simulink model "p2_d_sim"  (R2019a)
settings: Solver=VariableStepAuto  StartTime=0.0  StopTime=200  RelTol=1e-3
values from neighbouring files (symbols this model uses):
  a_phi1 = 2.87    [p2_d.m]    (also in p2_e.m)
  a_phi2 = -0.65    [p2_d.m]    (also in p2_e.m)
  k_dphi = k_d_phi    [p2_d.m]    (also in p2_e.m)
  k_g = g/V_g    (= 0.0608896551724)    [p2_d.m]    (also in p2_e.m)
  k_iphi = k_i_phi    (= -0.6)    [p2_d.m]    (also in p2_e.m)
  k_ix = k_i_chi    [p2_d.m]    (also in p2_e.m)
  k_pphi = k_p_phi    [p2_d.m]    (also in p2_e.m)
  k_px = k_p_chi    [p2_d.m]    (also in p2_e.m)
undefined symbols (not defined in the file or in its folder): sigbuilder_block
libraries: simulink_extras x2
settings Model: Creator=lenovo  LastModifiedBy=zhy

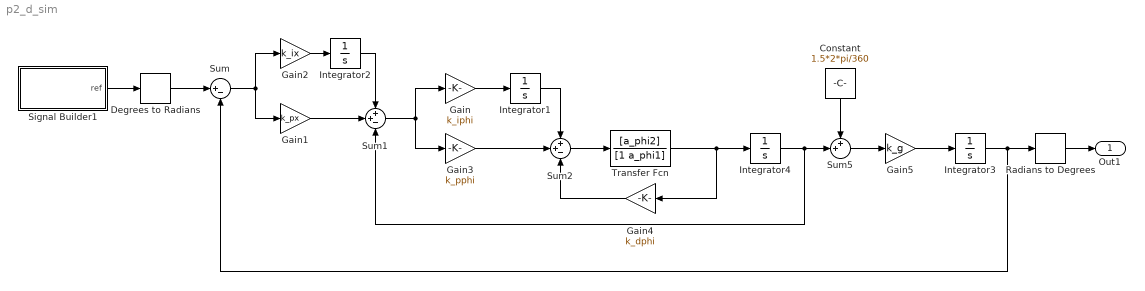
== system p2_d_sim ==
  Constant : Constant  Value=1.5*2*pi/360
  Degrees to Radians : simulink_extras/Transformations/Degrees to Radians
  Gain : Gain  Gain=k_iphi
  Gain1 : Gain  Gain=k_px
  Gain2 : Gain  Gain=k_ix
  Gain3 : Gain  Gain=k_pphi
  Gain4 : Gain  Gain=k_dphi
  Gain5 : Gain  Gain=k_g
  Integrator{1..4} (4 alike) : Integrator
  Radians to Degrees : simulink_extras/Transformations/Radians to Degrees
  Signal Builder1 : Subsystem  Tag=STV Subsys  LoadFcn=sigbuilder_block('load');  StartFcn=sigbuilder_block('start');  StopFcn=sigbuilder_block('stop');  ClipboardFcn=sigbuilder_block('clipboard');  mask(Sigbuilder block){tuvar=[0:10]}
      mask help: Simulink:masks:SigbuilderBlock_MD
      mask init:
      | if ~strcmp(get_param(bdroot(gcbh),'SimulationStatus'),'stopped') tuvar = sigbuilder_block('maskInit'); end
      settings: CopyFcn=sigbuilder_block('copy');  DeleteFcn=sigbuilder_block('delete');  ModelCloseFcn=sigbuilder_block('modelClose');  PreSaveFcn=sigbuilder_block('preSave');  PauseFcn=sigbuilder_block('pause');  ContinueFcn=sigbuilder_block('continue');  NameChangeFcn=sigbuilder_block('namechange');  OpenFcn=sigbuilder_block('open',[411 163.2 550.8 400.2 ]);  CloseFcn=sigbuilder_block('close');
      mask Display: plot(0, 0, 100, 100,[2, 2, 32, 32, 2], [68, 8, 8, 68, 68],[32, 2], [38, 38], [32, 19, 2],[53, 60, 44], [32, 17, 17, 2],[16, 16, 31, 31]);txt = getActiveGroup(gcbh);text(2, 100, txt,'verticalAlignment', 'top');
  Sum : Sum  Inputs=|+-
  Sum1 : Sum  Inputs=++-
  Sum2 : Sum  Inputs=++-
  Sum5 : Sum  Inputs=++|
  Transfer Fcn : TransferFcn  Numerator=[a_phi2]  Denominator=[1 a_phi1]
  Out1 : Outport
  wires:
  Sum/1 -> Gain1/1, Gain2/1
  Sum1/1 -> Gain3/1, Gain/1
  Sum5/1 -> Gain5/1
  Degrees to Radians/1 -> Sum/1
  Gain2/1 -> Integrator2/1
  Integrator2/1 -> Sum1/1
  Gain1/1 -> Sum1/2
  Gain/1 -> Integrator1/1
  Gain3/1 -> Sum2/2
  Transfer Fcn/1 -> Gain4/1, Integrator4/1
  Integrator4/1 -> Sum5/2, Sum1/3
  Constant/1 -> Sum5/1
  Integrator3/1 -> Radians to Degrees/1, Sum/2
  Gain5/1 -> Integrator3/1
  Signal Builder1/1(ref) -> Degrees to Radians/1
  Sum2/1 -> Transfer Fcn/1
  Gain4/1 -> Sum2/3
  Integrator1/1 -> Sum2/1
  Radians to Degrees/1 -> Out1/1

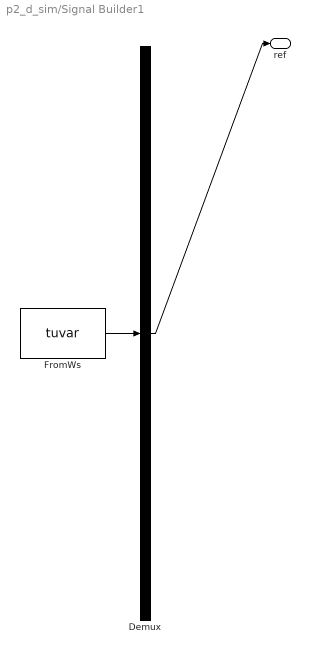
== system p2_d_sim/Signal Builder1 ==
  Demux : Demux  Tag=STV Demux  Outputs=1
  FromWs : FromWorkspace  Tag=STV FromWs  VariableName=tuvar  SampleTime=0
      SigBuilderData=|
      | common.afterFinalStr = 'Extrapolate'
      | common.sampleTime = 0
      | dataSet.timeRange = [0 200]
      | dataSet.name = 'Group 1'
      | sbobj.Groups.Name = 'Group 1'
      | sbobj.Groups.Signals.Name = 'ref'
      | sbobj.Groups.Signals.XData = [0 25 25 75 75 125 125 200]
      | sbobj.Groups.Signals.YData = [0 0 5 5 10 10 15 15]
      | sbobj.Groups.TimeRange = [0 200]
  ref : Outport  Tag=STV Outport
  wires:
  FromWs/1 -> Demux/1
  Demux/1 -> ref/1
